simulink model "T1_4_Pinon_Cremallera_Simulink"  (R2022b)
settings: Solver=VariableStepAuto  StartTime=0.0  StopTime=20  MaxStep=0.001  RelTol=1e-3
settings Model: Creator=miel_  LastModifiedBy=miel_

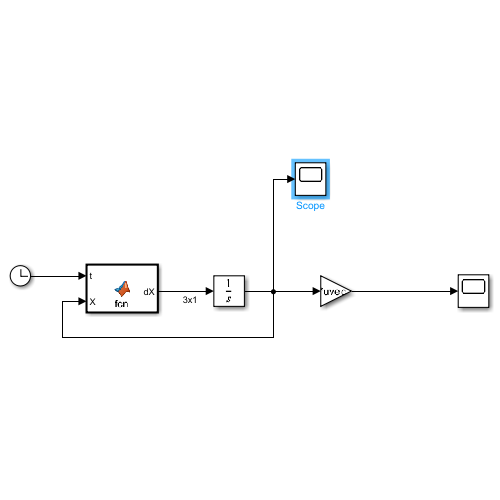
[thumbnail: Simulink's stored preview of the top-level diagram]
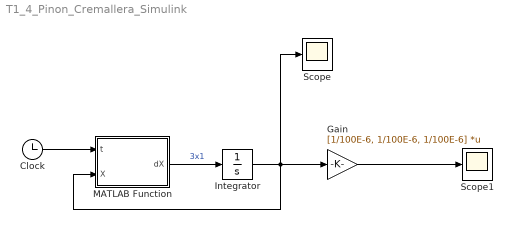
== system T1_4_Pinon_Cremallera_Simulink ==
  Clock : Clock
  Gain : Gain  Gain=[1/100E-6, 1/100E-6, 1/100E-6]  Multiplication=Matrix(K*u) (u vector)
  Integrator : Integrator  InitialCondition=[0; 0; 0]
  MATLAB Function : MATLAB Function  TreatAsAtomicUnit=on
  Scope : Scope
  Scope1 : Scope
  wires:
  MATLAB Function/1(dX) -> Integrator/1  "3x1"
  Integrator/1 -> MATLAB Function/2(X), Scope/1, Gain/1
  Gain/1 -> Scope1/1
  Clock/1 -> MATLAB Function/1(t)

== matlab function T1_4_Pinon_Cremallera_Simulink/MATLAB Function ==
  data: t input; dX output; X input
function dX = fcn(t, X)

% Parámetros del sistema

L=1E-3; R=10; J=0.001; B=0.2; k_t=1; k_b=1; n=10;
N=30; M=5; b=0.8; k=0.5;

dospienecuadrada = (2*pi*N)^2;
denominador = (J*(dospienecuadrada)+(n^2)*M);

% Matrices

A = [0, 0, n/(2*pi*N); 0, -R/L, -k_b/L; -(n*k*2*pi*N)/denominador, (k_t*dospienecuadrada)/denominador, -((B*dospienecuadrada)+((n^2)*b))/denominador];
B = [0; 1/L; 0];

% U = 0;
U = 2;
% U = 2*sin(100*t);

dX = A*X + B*U;
